simulink model "HW6_pblm3"  (R2020b)
settings: Solver=VariableStepAuto  StartTime=0.0  StopTime=10.0  RelTol=1e-3
values from neighbouring files (symbols this model uses):
  K = toeplitz([0, -1, 0],[0, 0, -1])    [MECH6313_HW6_pblm3.m]
settings Model: Creator=Jonas  LastModifiedBy=Jonas

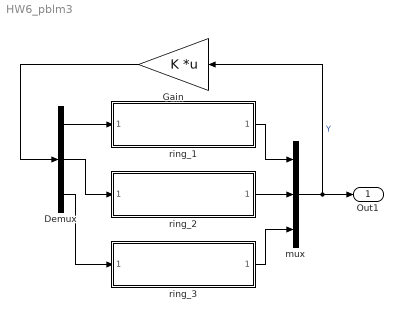
== system HW6_pblm3 ==
  Demux : Demux  Outputs=3
  Gain : Gain  Gain=K  Multiplication=Matrix(K*u) (u vector)
  mux : Mux  Inputs=3
  ring_1 : Subsystem  ReferencedSubsystem=ring_oscillator_stage  tau=tau1  alpha=alpha1  beta=beta1  x0=x01
  ring_2 : Subsystem  ReferencedSubsystem=ring_oscillator_stage  tau=tau2  alpha=alpha2  beta=beta2  x0=x02
  ring_3 : Subsystem  ReferencedSubsystem=ring_oscillator_stage  tau=tau3  alpha=alpha3  beta=beta3  x0=x03
  Out1 : Outport
  wires:
  Demux/1 -> ring_1/1
  Gain/1 -> Demux/1
  Demux/2 -> ring_2/1
  Demux/3 -> ring_3/1
  ring_3/1 -> mux/3
  ring_2/1 -> mux/2
  ring_1/1 -> mux/1
  mux/1 -> Out1/1, Gain/1  "Y"
